simulink model "bldc_test_01"  (R2020b)
settings: Solver=ode23tb  StartTime=0.0  StopTime=2  MaxStep=0.02  RelTol=1e-3
libraries: powerlib x9
settings Model: Creator=MSI  LastModifiedBy=macbook
settings DataIOCC: ReturnWorkspaceOutputs=off
settings OptimizationCC: LifeSpan=inf
settings DebuggingCC: ArithmeticOperatorsInVariantConditions=warning
settings SFSimCC: SimUseLocalCustomCode=off  CustomCodeUndefinedFunction=UseInterfaceOnly
settings RTWCC: RTWUseLocalCustomCode=off
settings CodeAppCC: StateflowObjectComments=on

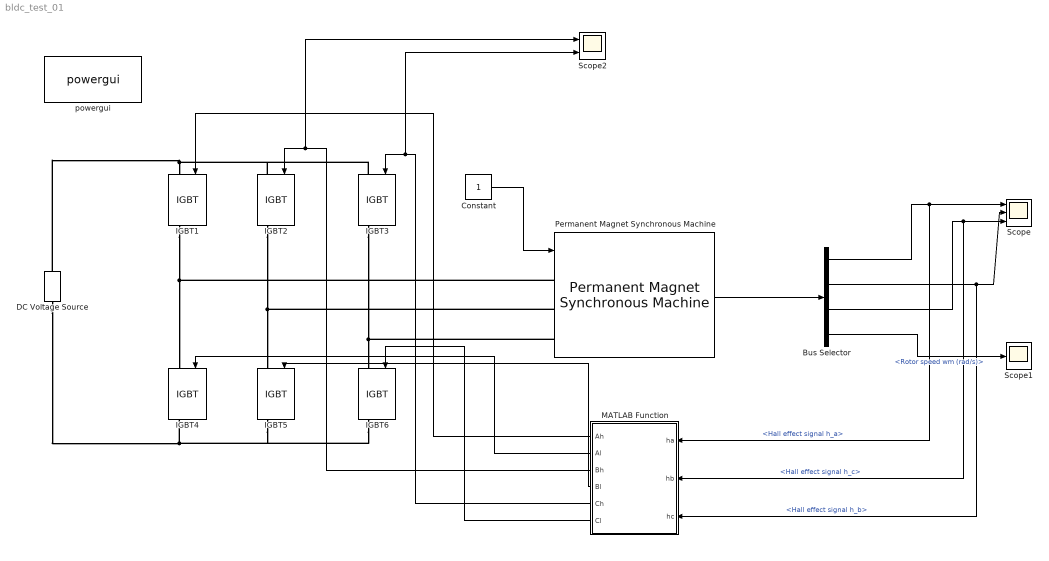
== system bldc_test_01 ==
  Bus Selector : BusSelector  OutputSignals=Hall effect signal h_a,Hall effect signal h_b,Hall effect signal h_c,Rotor speed wm (rad/s)
  Constant : Constant
  DC Voltage Source : powerlib/Electrical Sources/DC Voltage Source  Amplitude=64  Measurements=None
  IGBT{1..6} (6 alike) : powerlib/Power Electronics/IGBT  Ron=0.001  Lon=0  Vf=1  Tf=1e-6  Tt=2e-6  IC=0  Rs=1e5  Cs=inf  Measurements=on
  MATLAB Function : MATLAB Function  TreatAsAtomicUnit=on
  Permanent Magnet Synchronous Machine : powerlib/Machines/Permanent Magnet Synchronous Machine  NbPhases=3  FluxDistribution=Sinusoidal  RotorType=Round  MechanicalLoad=Torque Tm  PresetModel=No  ShowDetailedParameters=on  MeasurementBus=off  Resistance=0.0485  Inductance=8.5e-3  dqInductances=[8.5e-3,8.5e-3]  La=0.000395  MachineConstant=Flux linkage established by magnets (V.s)  Flux=0.1194  VoltageCst=86.6271  TorqueCst=0.7164  Flat=120  Mechanical=[0.0027 0.0004924 4 0]  PolePairs=4  InitialConditions=[0,0, 0,0]  InitialConditions5ph=[0 0 0 0 0 0]  RefAngle=90 degrees behind phase A axis (modified Park)  IterativeDiscreteModel=Trapezoidal non iterative  TsBlock=-1  TsPowergui=0
  Scope : Scope  NumInputPorts=3
  Scope1 : Scope
  Scope2 : Scope  NumInputPorts=2
  powergui : powerlib/powergui  Priority=1  SimulationMode=Continuous  SampleTime=50e-6  frequency=60  Iterations=50  frequencyindice=0  Pbase=100e6  ErrMax=1e-4  UnitsV=kV  UnitsW=MW  buscounter=0  FunctionMessages=off  echomessages=off  EnableUseOfTLC=off  CurrentSourceSwitches=off  DisableSnubberDevices=off  DisableRonSwitches=off  DisableVfSwitches=off  DisplayEquations=off  AutomaticDiscreteSolvers=off  SolverType=Tustin/Backward Euler (TBE)  Interpol=off  ExternalGateDelay=off  methode=off  Ts=100  x0status=blocks  SPID=on  SwTol=0  HookPort=off  NonlinearTolerance=1e-4  nMaxIteration=100  ContinueOnMaxIteration=off  RestoreLinks=warning  ResistiveCurrentMeasurement=off  Frange=[0:2:500]  Ylog=off  Xlog=on  ShowGrid=off  save=off  variable=ZData  structure=0  ZoomFFT=off  StartTime=0.0  cycles=1  DisplayStyle=1  fundamental=60  FreqAxis=off  MaxFrequency=1000  frequencyindicesteady=1  RmsSteady=1  display=off
  wires:
  Constant/1 -> Permanent Magnet Synchronous Machine/1
  MATLAB Function/1(Ah) -> IGBT1/1
  MATLAB Function/2(Al) -> IGBT4/1
  MATLAB Function/3(Bh) -> Scope2/1, IGBT2/1
  MATLAB Function/4(Bl) -> IGBT5/1
  MATLAB Function/5(Ch) -> Scope2/2, IGBT3/1
  MATLAB Function/6(Cl) -> IGBT6/1
  Permanent Magnet Synchronous Machine/1 -> Bus Selector/1
  Bus Selector/1 -> MATLAB Function/1(ha), Scope/1  "<Hall effect signal h_a>"
  Bus Selector/2 -> MATLAB Function/3(hc), Scope/2  "<Hall effect signal h_b>"
  Bus Selector/3 -> MATLAB Function/2(hb), Scope/3  "<Hall effect signal h_c>"
  Bus Selector/4 -> Scope1/1  "<Rotor speed wm (rad/s)>"
  connections:
  DC Voltage Source/RConn1 -- IGBT2/LConn1 -- IGBT3/LConn1 -- IGBT1/LConn1
  DC Voltage Source/LConn1 -- IGBT6/RConn1 -- IGBT5/RConn1 -- IGBT4/RConn1
  IGBT1/RConn1 -- Permanent Magnet Synchronous Machine/LConn1 -- IGBT4/LConn1
  IGBT2/RConn1 -- Permanent Magnet Synchronous Machine/LConn2 -- IGBT5/LConn1
  IGBT3/RConn1 -- Permanent Magnet Synchronous Machine/LConn3 -- IGBT6/LConn1

== matlab function bldc_test_01/MATLAB Function ==
  data: ha input; Ah output; hb input; hc input; Al output; Bh output; Bl output; Ch output; Cl output
function [Ah,Al,Bh,Bl,Ch,Cl] = fcn(ha,hb,hc) 
 
% 000 
if (ha==0)&&(hb==0)&&(hc==0) 
    Ah=0;Al=0; 
    Bh=0;Bl=0; 
    Ch=0;Cl=0; 
% 110 
elseif (ha==1)&&(hb==1)&&(hc==0) 
    Ah=0;Al=0; 
    Bh=1;Bl=0; 
    Ch=0;Cl=1; 
 
% 010 
elseif (ha==0)&&(hb==1)&&(hc==0) 
    Ah=0;Al=1; 
    Bh=1;Bl=0; 
    Ch=0;Cl=0; 
 
% 011 
elseif (ha==0)&&(hb==1)&&(hc==1) 
    Ah=0;Al=1; 
    Bh=0;Bl=0; 
    Ch=1;Cl=0; 
 
% 001 
elseif (ha==0)&&(hb==0)&&(hc==1) 
    Ah=0;Al=0; 
    Bh=0;Bl=1; 
    Ch=1;Cl=0; 
 
% 101 
elseif (ha==1)&&(hb==0)&&(hc==1) 
    Ah=1;Al=0; 
    Bh=0;Bl=1; 
    Ch=0;Cl=0; 
 
% 100 
elseif (ha==1)&&(hb==0)&&(hc==0) 
    Ah=1;Al=0; 
    Bh=0;Bl=0; 
    Ch=0;Cl=1; 
% 111 
elseif (ha==1)&&(hb==1)&&(hc==1) 
    Ah=0;Al=0; 
    Bh=0;Bl=0; 
    Ch=0;Cl=0; 
else 
    Ah=0;Al=0; 
    Bh=0;Bl=0; 
    Ch=0;Cl=0; 
end 
 
end
